simulink model "fcs_lab_05_model_02"  (R2014b)
settings: Solver=ode45  StartTime=0.0  StopTime=500  RelTol=1e-3
values from neighbouring files (symbols this model uses):
  C = 10    [fcs_lab_05_model_02_test.m]    (also in fcs_lab_05_model_03_test.m)
  e = 60    [fcs_lab_05_model_02_test.m]    (also in fcs_lab_05_model_03_test.m)
  L = 1    [fcs_lab_05_model_02_test.m]
  R = 10    [fcs_lab_05_model_02_test.m]
settings Model: Creator=Mashkoor Ahmed  LastModifiedBy=Mashkoor Ahmed

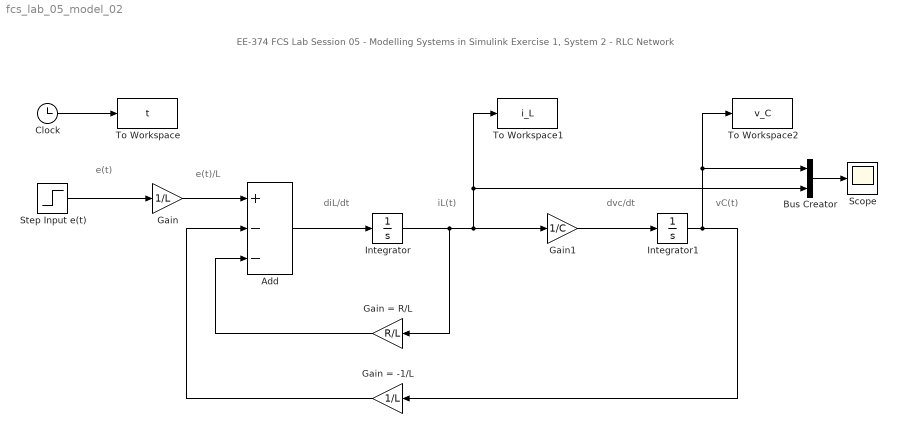
== system fcs_lab_05_model_02 ==
  note: EE-374 FCS Lab Session 05 - Modelling Systems in Simulink
      | Exercise 1, System 2 - RLC Network
  note: vC(t)
  note: dvc/dt
  note: iL(t)
  note: diL/dt
  note: e(t)/L
  note: e(t)
  Add : Sum  Inputs=+--
  Bus Creator : BusCreator  Inputs=2
  Clock : Clock
  Gain : Gain  Gain=1/L
  Gain = -1/L : Gain  Gain=1/L
  Gain = R/L : Gain  Gain=R/L
  Gain1 : Gain  Gain=1/C
  Integrator : Integrator
  Integrator1 : Integrator
  Scope : Scope
  Step Input e(t) : Step  Time=0  After=e  SampleTime=0
  To Workspace : ToWorkspace  VariableName=t  SampleTime=-1
  To Workspace1 : ToWorkspace  VariableName=i_L  SampleTime=-1
  To Workspace2 : ToWorkspace  VariableName=v_C  SampleTime=-1
  wires:
  Step Input e(t)/1 -> Gain/1
  Gain/1 -> Add/1
  Add/1 -> Integrator/1
  Gain = R/L/1 -> Add/3
  Integrator/1 -> Bus Creator/2, To Workspace1/1, Gain1/1, Gain = R/L/1
  Gain = -1/L/1 -> Add/2
  Gain1/1 -> Integrator1/1
  Integrator1/1 -> Bus Creator/1, To Workspace2/1, Gain = -1/L/1
  Clock/1 -> To Workspace/1
  Bus Creator/1 -> Scope/1
